simulink library "amplitude_spectrum"  (Simulink 9.2)
settings: Solver=ode45  StartTime=0.0  StopTime=10.0  RelTol=1e-3  EnableMultiTasking=on
libraries: dspspect3 x1, dspsigops x1
settings Model: Creator=Administrator  LastModifiedBy=rmirr

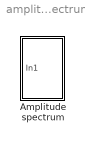
== system amplitude_spectrum ==
  Amplitude spectrum : Subsystem  mask(Amplitude Spectrum){}
      mask help:
      | This component takes periodic signal as input and display its amplitud spectrum.
      |
      | Input signal frequency range (0, 50000] Hz.
      mask Help:
      | Sampling frequency is 1e5 Hz. Need to change this parameter to include high frequency components in the results. It should be 2 times of the frequency of the highest frequency component.
      | FFT is 4096 points.

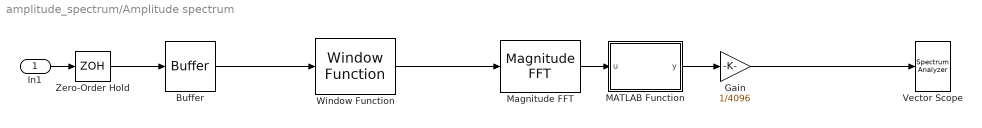
== system amplitude_spectrum/Amplitude spectrum ==
  In1 : Inport
  Buffer : Buffer  N=4096
  Gain : Gain  Gain=1/4096
  MATLAB Function : MATLAB Function  TreatAsAtomicUnit=on
  Magnitude FFT : dspspect3/Magnitude FFT  mag_or_magsq=Magnitude  FFTImplementation=Auto  fftLenInherit=on  fftsize=1024  WrapInput=on
      settings: SourceProductName=DSP System Toolbox  SourceProductBaseCode=DS
  Vector Scope : SpectrumAnalyzer
  Window Function : dspsigops/Window Function  winmode=Apply window to input  wintype=Boxcar  sampmode=Continuous  samptime=1  N=64  Rs=50  beta=10  winsamp=Periodic  UserWindow=flattopwin  OptParams=on  UserParams={'periodic'}  dataType=double  isSigned=on  wordLen=16  udDataType=sfix(16)  fracBitsMode=Best precision  numFracBits=15  roundingMode=Floor  overflowMode=off  numSidelobes=4  sidelobeLevel=-30
      settings: SourceProductName=DSP System Toolbox  SourceProductBaseCode=DS
  Zero-Order Hold : ZeroOrderHold  SampleTime=1/2e5
  wires:
  Zero-Order Hold/1 -> Buffer/1
  Magnitude FFT/1 -> MATLAB Function/1(u)
  Gain/1 -> Vector Scope/1
  Buffer/1 -> Window Function/1
  Window Function/1 -> Magnitude FFT/1
  In1/1 -> Zero-Order Hold/1
  MATLAB Function/1(y) -> Gain/1

== matlab function Amplitude spectrum/MATLAB Function ==
  data: u input double; y output double
function y = fcn(u)

y = fftshift(u);
